simulink model "seminar5_topic22"  (R2018b)
settings: Solver=VariableStepAuto  StartTime=0.0  StopTime=0.08  RelTol=1e-3
values from neighbouring files (symbols this model uses):
  tem1 = i    [S5_analysis.m]
  tem2 = 100 - i    [S5_analysis.m]
  tem3 = 1e-3.*(i./100)    [S5_analysis.m]
libraries: powerlib x9, powerlib_meascontrol x8
settings Model: Creator=96547  LastModifiedBy=Administrator

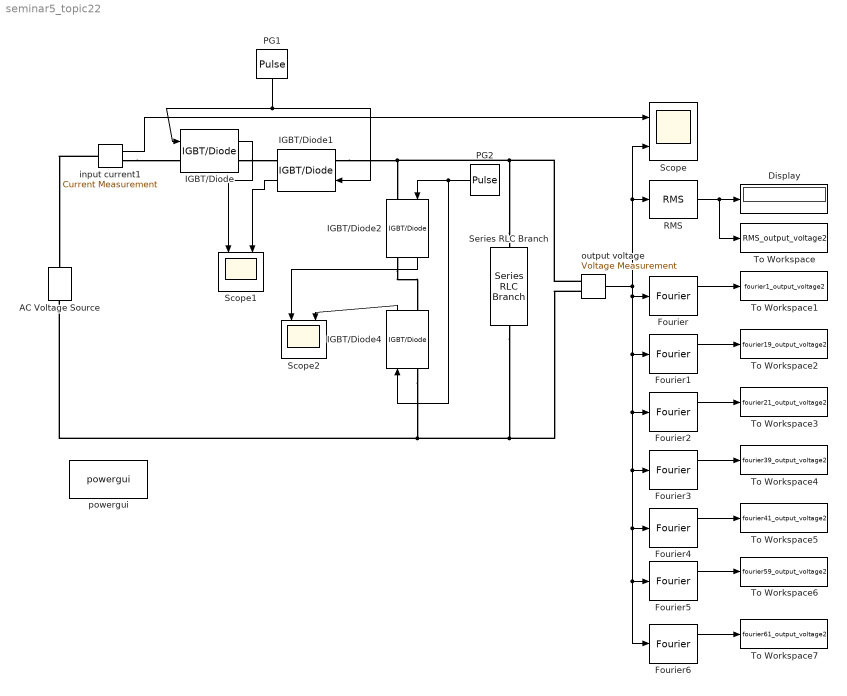
== system seminar5_topic22 ==
  AC Voltage Source : powerlib/Electrical Sources/AC Voltage Source  Amplitude=220*sqrt(2)  Phase=0  Frequency=50  SampleTime=0  Measurements=None  BusType=swing  Pref=10e3  Qref=0  Qmin=-inf  Qmax=+inf
      settings: SourceProductName=Simscape Electrical
  Display : Display
  Fourier : powerlib_meascontrol/Measurements/Fourier  Freq=50  n=1  InInit=[0, 0]  Ts=0
      settings: SourceProductName=Simscape Power Systems
  Fourier1 : powerlib_meascontrol/Measurements/Fourier  Freq=50  n=19  InInit=[0, 0]  Ts=0
      settings: SourceProductName=Simscape Power Systems
  Fourier2 : powerlib_meascontrol/Measurements/Fourier  Freq=50  n=21  InInit=[0, 0]  Ts=0
      settings: SourceProductName=Simscape Power Systems
  Fourier3 : powerlib_meascontrol/Measurements/Fourier  Freq=50  n=39  InInit=[0, 0]  Ts=0
      settings: SourceProductName=Simscape Power Systems
  Fourier4 : powerlib_meascontrol/Measurements/Fourier  Freq=50  n=41  InInit=[0, 0]  Ts=0
      settings: SourceProductName=Simscape Power Systems
  Fourier5 : powerlib_meascontrol/Measurements/Fourier  Freq=50  n=59  InInit=[0, 0]  Ts=0
      settings: SourceProductName=Simscape Power Systems
  Fourier6 : powerlib_meascontrol/Measurements/Fourier  Freq=50  n=61  InInit=[0, 0]  Ts=0
      settings: SourceProductName=Simscape Power Systems
  IGBT/Diode{,1..2,4} (4 alike) : powerlib/Power Electronics/IGBT//Diode  Ron=1e-3  Rs=1e5  Cs=inf  Measurements=on
      settings: SourceProductName=Simscape Electrical
  PG1 : DiscretePulseGenerator  PulseType=Time based  Period=1e-3  PulseWidth=tem1
  PG2 : DiscretePulseGenerator  PulseType=Time based  Period=1e-3  PulseWidth=tem2  PhaseDelay=tem3
  RMS : powerlib_meascontrol/Measurements/RMS  TrueRMS=on  Freq=60  RMSInit=120  Ts=0
      settings: SourceProductName=Simscape Electrical
  Scope : Scope  NumInputPorts=2
  Scope1 : Scope  NumInputPorts=2
  Scope2 : Scope  NumInputPorts=2
  Series RLC Branch : powerlib/Elements/Series RLC Branch  LConnTagsString=__new0  RConnTagsString=__new0  BranchType=RL  Resistance=10  Inductance=2.2e-3  SetiL0=off  InitialCurrent=0  Capacitance=1e-6  Setx0=off  InitialVoltage=0  Measurements=None
      settings: SourceProductName=Simscape Electrical
  To Workspace : ToWorkspace  VariableName=RMS_output_voltage2  SampleTime=-1
      settings: Save2DSignal=2-D array (concatenate along first dimension)
  To Workspace1 : ToWorkspace  VariableName=fourier1_output_voltage2  SampleTime=-1
      settings: Save2DSignal=2-D array (concatenate along first dimension)
  To Workspace2 : ToWorkspace  VariableName=fourier19_output_voltage2  SampleTime=-1
      settings: Save2DSignal=2-D array (concatenate along first dimension)
  To Workspace3 : ToWorkspace  VariableName=fourier21_output_voltage2  SampleTime=-1
      settings: Save2DSignal=2-D array (concatenate along first dimension)
  To Workspace4 : ToWorkspace  VariableName=fourier39_output_voltage2  SampleTime=-1
      settings: Save2DSignal=2-D array (concatenate along first dimension)
  To Workspace5 : ToWorkspace  VariableName=fourier41_output_voltage2  SampleTime=-1
      settings: Save2DSignal=2-D array (concatenate along first dimension)
  To Workspace6 : ToWorkspace  VariableName=fourier59_output_voltage2  SampleTime=-1
      settings: Save2DSignal=2-D array (concatenate along first dimension)
  To Workspace7 : ToWorkspace  VariableName=fourier61_output_voltage2  SampleTime=-1
      settings: Save2DSignal=2-D array (concatenate along first dimension)
  input current1 : powerlib/Measurements/Current Measurement  PhasorSimulation=off  OutputType=Complex  PSBequivalent=0
      settings: SourceProductName=Simscape Electrical
  output voltage : powerlib/Measurements/Voltage Measurement  PhasorSimulation=off  OutputType=Complex  PSBequivalent=0
      settings: SourceProductName=Simscape Electrical
  powergui : powerlib/powergui  Priority=1  SimulationMode=Continuous  SampleTime=50e-6  frequency=60  Iterations=50  frequencyindice=50  Pbase=100e6  ErrMax=1e-4  UnitsV=kV  UnitsW=MW  buscounter=0  FunctionMessages=off  echomessages=off  EnableUseOfTLC=off  CurrentSourceSwitches=off  DisableSnubberDevices=off  DisableRonSwitches=off  DisableVfSwitches=off  DisplayEquations=off  SolverType=Tustin/Backward Euler (TBE)  Interpol=off  ExternalGateDelay=off  methode=off  Ts=100  x0status=blocks  SPID=on  SwTol=0  HookPort=off  RestoreLinks=warning  ResistiveCurrentMeasurement=off  Frange=[0:2:500]  Ylog=off  Xlog=on  ShowGrid=off  save=off  variable=ZData  structure=ScopeData  ZoomFFT=on  StartTime=0  cycles=4  DisplayStyle=1  fundamental=50  FreqAxis=off  MaxFrequency=6000  frequencyindicesteady=1  RmsSteady=1  display=off
  wires:
  output voltage/1 -> RMS/1, Scope/2, Fourier6/1, Fourier5/1, Fourier4/1, Fourier3/1, Fourier2/1, Fourier1/1, Fourier/1
  RMS/1 -> To Workspace/1, Display/1
  PG1/1 -> IGBT/Diode/1, IGBT/Diode1/1
  PG2/1 -> IGBT/Diode2/1, IGBT/Diode4/1
  input current1/1 -> Scope/1
  IGBT/Diode/1 -> Scope1/1
  IGBT/Diode1/1 -> Scope1/2
  IGBT/Diode2/1 -> Scope2/1
  IGBT/Diode4/1 -> Scope2/2
  Fourier/1 -> To Workspace1/1
  Fourier6/1 -> To Workspace7/1
  Fourier5/1 -> To Workspace6/1
  Fourier4/1 -> To Workspace5/1
  Fourier3/1 -> To Workspace4/1
  Fourier2/1 -> To Workspace3/1
  Fourier1/1 -> To Workspace2/1
  connections:
  Series RLC Branch/LConn1 -- output voltage/LConn1 -- IGBT/Diode1/LConn1 -- IGBT/Diode2/LConn1
  Series RLC Branch/RConn1 -- output voltage/LConn2 -- AC Voltage Source/LConn1 -- IGBT/Diode4/LConn1
  IGBT/Diode/RConn1 -- IGBT/Diode1/RConn1
  IGBT/Diode2/RConn1 -- IGBT/Diode4/RConn1
  input current1/RConn1 -- IGBT/Diode/LConn1
  input current1/LConn1 -- AC Voltage Source/RConn1
